simulink model "motorDistCtrl_soln"  (R2017a)
settings: Solver=VariableStepAuto  StartTime=0.0  StopTime=10.0  RelTol=1e-3
PreLoadFcn:
  | robotParameters;
values from neighbouring files (symbols this model uses):
  ticksPerRot = 627.2    [robotParameters.m]
  wheelR = 0.052    [robotParameters.m]
undefined symbols (not defined in the file or in its folder): motorIp, motorSp
libraries: mobileRoboticsTrainingLib x2, simulink x1
settings Model: Creator=sseshadr  LastModifiedBy=shiremat

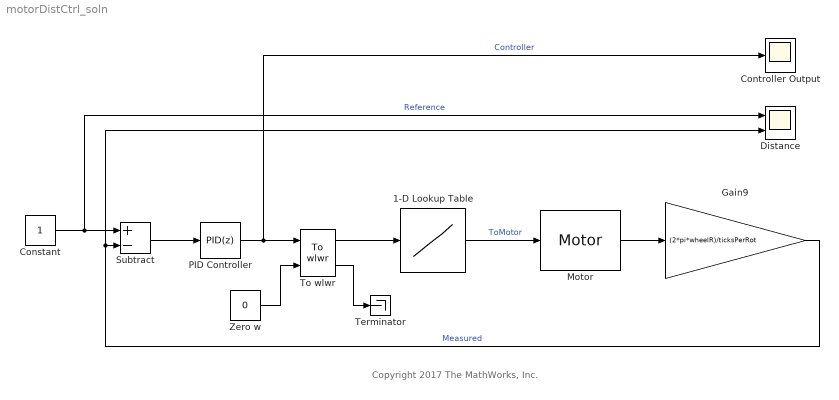
== system motorDistCtrl_soln ==
  note: Copyright 2017 The MathWorks, Inc.
  1-D Lookup Table : Lookup_n-D  NumberOfTableDimensions=1  BreakpointsForDimension1=motorSp  Table=motorIp  ExtrapMethod=Clip  InternalRulePriority=Speed  RndMeth=Simplest  InputSameDT=on
  Constant : Constant
  Controller Output : Scope
  Distance : Scope  NumInputPorts=2
  Gain9 : Gain  Gain=(2*pi*wheelR)/ticksPerRot
  Motor : mobileRoboticsTrainingLib/Motor  motorPlant=wheelMotorModel  sensorType=Position
      settings: SourceProductName=Mobile Robotics Training Library
  PID Controller : simulink/Continuous/PID Controller  Controller=PID  TimeDomain=Discrete-time  SampleTime=-1  IntegratorMethod=Forward Euler  FilterMethod=Forward Euler  Form=Parallel  UseFilter=on  ControllerParametersSource=internal  P=8.84600617438508  I=0.42540687501944  D=-0.0140783779685636  N=151.701833251505  InitialConditionSource=internal  InitialConditionForIntegrator=0  InitialConditionForFilter=0  ExternalReset=none  LimitOutput=on  UpperSaturationLimit=0.6  LowerSaturationLimit=-0.6  LinearizeAsGain=on  AntiWindupMode=clamping  Kb=1  TrackingMode=off  Kt=1  PParamMin=[]  PParamMax=[]  IParamMin=[]  IParamMax=[]  DParamMin=[]  DParamMax=[]  NParamMin=[]  NParamMax=[]  KbParamMin=[]  KbParamMax=[]  KtParamMin=[]  KtParamMax=[]  POutMin=[]  POutMax=[]  IOutMin=[]  IOutMax=[]  DOutMin=[]  DOutMax=[]  NOutMin=[]  NOutMax=[]  KbOutMin=[]  KbOutMax=[]  KtOutMin=[]  KtOutMax=[]  IntegratorOutMin=[]  IntegratorOutMax=[]  FilterOutMin=[]  FilterOutMax=[]  SumOutMin=[]  SumOutMax=[]  SumI1OutMin=[]  SumI1OutMax=[]  SumI2OutMin=[]  SumI2OutMax=[]  SumI3OutMin=[]  SumI3OutMax=[]  SumDOutMin=[]  SumDOutMax=[]  SaturationOutMin=[]  SaturationOutMax=[]  IntegratorContinuousStateAttributes=''  IntegratorStateMustResolveToSignalObject=off  IntegratorRTWStateStorageClass=Auto  FilterContinuousStateAttributes=''  FilterStateMustResolveToSignalObject=off  FilterRTWStateStorageClass=Auto  DifferentiatorICPrevScaledInput=0  DifferentiatorOutMin=[]  DifferentiatorOutMax=[]  InitialConditionSetting=Output
  Subtract : Sum  Inputs=+-
  Terminator : Terminator
  To wlwr : mobileRoboticsTrainingLib/To wlwr  axleLength=axleLength  wheelR=wheelR
  Zero w : Constant  Value=0
  wires:
  Constant/1 -> Distance/1, Subtract/1  "Reference"
  Gain9/1 -> Distance/2, Subtract/2  "Measured"
  To wlwr/1 -> 1-D Lookup Table/1
  Zero w/1 -> To wlwr/2
  To wlwr/2 -> Terminator/1
  PID Controller/1 -> Controller Output/1, To wlwr/1  "Controller"
  1-D Lookup Table/1 -> Motor/1  "ToMotor"
  Motor/1 -> Gain9/1
  Subtract/1 -> PID Controller/1
